simulink model "es1_dist"  (R2014a)
settings: Solver=ode45  StartTime=0.0  StopTime=20.0  RelTol=1e-3
values from neighbouring files (symbols this model uses):
  Kc = 5    [es1.m]
  Kr = 1    [es1.m]
  Rd = (1 + taud*s) / (1 + taud*s/md)    [es1.m]
  Ri = (1 + taui*s/mi) / (1 + taui*s)    [es1.m]
  s = tf('s')    [es1.m]
libraries: cstblocks x2
settings Model: Creator=HP  LastModifiedBy=HP

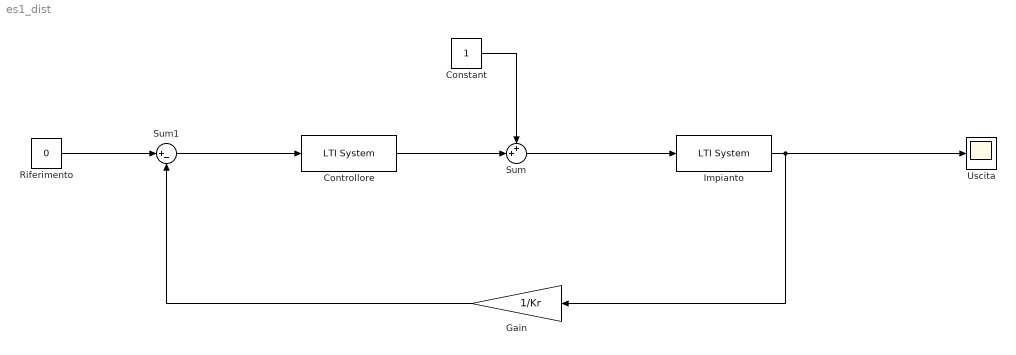
== system es1_dist ==
  Constant : Constant
  Controllore : cstblocks/LTI System  sys=Kc*Rd^2*Ri^2/s  IC=[]
  Gain : Gain  Gain=1/Kr
  Impianto : cstblocks/LTI System  sys=F  IC=[]
  Riferimento : Constant  Value=0
  Sum : Sum  Inputs=++|
  Sum1 : Sum  Inputs=|+-
  Uscita : Scope
  wires:
  Controllore/1 -> Sum/2
  Sum/1 -> Impianto/1
  Sum1/1 -> Controllore/1
  Gain/1 -> Sum1/2
  Riferimento/1 -> Sum1/1
  Constant/1 -> Sum/1
  Impianto/1 -> Uscita/1, Gain/1
